simulink library "NNodeTether_cl"  (R2018b)
settings: Solver=VariableStepAuto  StartTime=0.0  StopTime=10.0  RelTol=1e-3
undefined symbols (not defined in the file): ini_Ri_o, ini_Vi_o, thr
libraries: tetherBuoyancyAndWeightNGreater2_ul x1, tetherInternalForcesNGreater2_ul x1, tetherDragForceNGreater2_ul x1
settings Model: Creator=asiddiq2  LastModifiedBy=mcobb

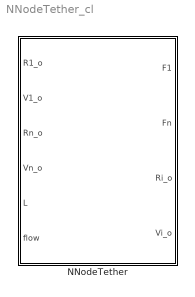
== system NNodeTether_cl ==
  NNodeTether : Subsystem

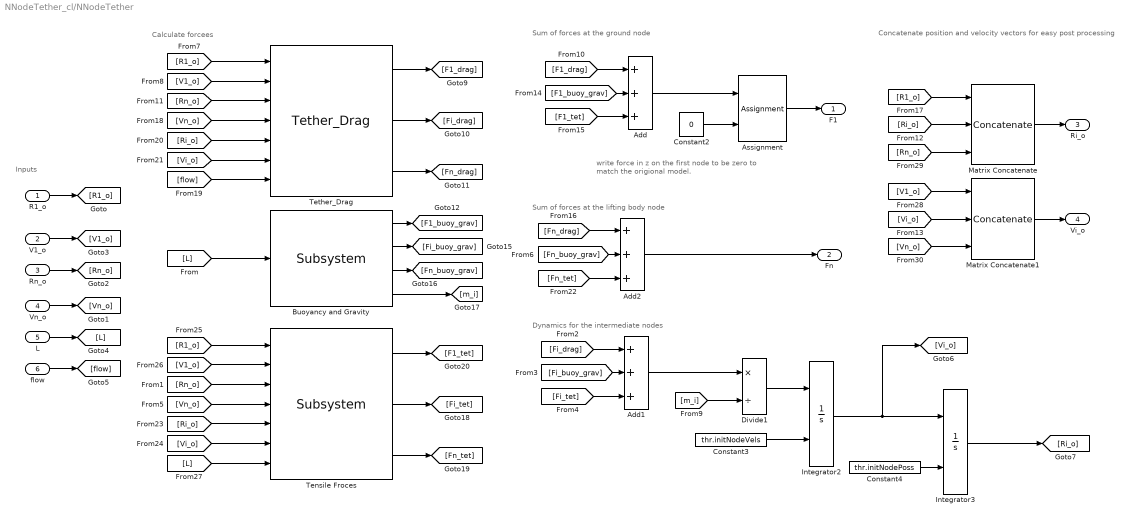
== system NNodeTether_cl/NNodeTether ==
  note: Concatenate position and velocity vectors for easy
      | post processing
  note: Calculate forcees
  note: Sum of forces at the lifting body node
  note: Dynamics for the intermediate nodes
  note: Sum of forces at the ground node
  note: write force in z on the first node to be zero
      | to match the origional model.
  note: Inputs
  R1_o : Inport
  V1_o : Inport  Port=2
  Rn_o : Inport  Port=3
  Vn_o : Inport  Port=4
  L : Inport  Port=5
  flow : Inport  Port=6
  Add : Sum  Inputs=+++
  Add1 : Sum  Inputs=+++
  Add2 : Sum  Inputs=+++
  Assignment : Assignment  NumberOfDimensions=2  DiagnosticForDimensions=Warning  IndexOptions=Index vector (dialog),Index vector (dialog)  Indices=3,1  OutputSizes=1,1
  Buoyancy and Gravity : tetherBuoyancyAndWeightNGreater2_ul/Subsystem  N=thr.N  dia_t=thr.diameter  rho_fluid=thr.fluidDensity  rho_tether=thr.density  g=thr.gravAccel
  Constant2 : Constant  Value=0
  Constant3 : Constant  Value=thr.initNodeVels
  Constant4 : Constant  Value=thr.initNodePoss
  Divide1 : Product  Inputs=*/
  Integrator2 : Integrator  InitialConditionSource=external  InitialCondition=ini_Vi_o
  Integrator3 : Integrator  InitialConditionSource=external  InitialCondition=ini_Ri_o
  Matrix Concatenate : Concatenate  NumInputs=3  Mode=Multidimensional array  ConcatenateDimension=2
  Matrix Concatenate1 : Concatenate  NumInputs=3  Mode=Multidimensional array  ConcatenateDimension=2
  Tensile Froces : tetherInternalForcesNGreater2_ul/Subsystem  N=thr.N  E=thr.youngsMod  dia_t=thr.diameter  mass=thr.vehicleMass  zeta=thr.dampingRatio
  Tether_Drag : tetherDragForceNGreater2_ul/Tether_Drag  Cd=thr.dragCoeff  rho_fluid=thr.fluidDensity  dia_t=thr.diameter
  F1 : Outport
  Fn : Outport  Port=2
  Ri_o : Outport  Port=3
  Vi_o : Outport  Port=4
  wires:
  R1_o/1 -> [R1_o]
  V1_o/1 -> [V1_o]
  Rn_o/1 -> [Rn_o]
  Vn_o/1 -> [Vn_o]
  L/1 -> [L]
  flow/1 -> [flow]
  [L] -> Buoyancy and Gravity/1
  [F1_buoy_grav] -> Add/2
  [F1_drag] -> Add/1
  [F1_tet] -> Add/3
  Assignment/1 -> F1/1
  Add/1 -> Assignment/1
  Constant2/1 -> Assignment/2
  Tether_Drag/1 -> [F1_drag]
  Tether_Drag/2 -> [Fi_drag]
  Tether_Drag/3 -> [Fn_drag]
  Buoyancy and Gravity/1 -> [F1_buoy_grav]
  Buoyancy and Gravity/2 -> [Fi_buoy_grav]
  Buoyancy and Gravity/3 -> [Fn_buoy_grav]
  Buoyancy and Gravity/4 -> [m_i]
  Tensile Froces/2 -> [Fi_tet]
  Tensile Froces/3 -> [Fn_tet]
  Tensile Froces/1 -> [F1_tet]
  [Fi_buoy_grav] -> Add1/2
  [Fi_tet] -> Add1/3
  [Fi_drag] -> Add1/1
  Add1/1 -> Divide1/1
  [m_i] -> Divide1/2
  Divide1/1 -> Integrator2/1
  Constant3/1 -> Integrator2/2
  Integrator2/1 -> [Vi_o], Integrator3/1
  Constant4/1 -> Integrator3/2
  Integrator3/1 -> [Ri_o]
  [Fn_drag] -> Add2/1
  [Fn_buoy_grav] -> Add2/2
  [Fn_tet] -> Add2/3
  Add2/1 -> Fn/1
  [R1_o] -> Tether_Drag/1
  [V1_o] -> Tether_Drag/2
  [Rn_o] -> Tether_Drag/3
  [Vn_o] -> Tether_Drag/4
  [Ri_o] -> Tether_Drag/5
  [Vi_o] -> Tether_Drag/6
  [flow] -> Tether_Drag/7
  [R1_o] -> Tensile Froces/1
  [Vn_o] -> Tensile Froces/4
  [Rn_o] -> Tensile Froces/3
  [Vi_o] -> Tensile Froces/6
  [Ri_o] -> Tensile Froces/5
  [V1_o] -> Tensile Froces/2
  [L] -> Tensile Froces/7
  [Rn_o] -> Matrix Concatenate/3
  [Ri_o] -> Matrix Concatenate/2
  [R1_o] -> Matrix Concatenate/1
  Matrix Concatenate/1 -> Ri_o/1
  [V1_o] -> Matrix Concatenate1/1
  Matrix Concatenate1/1 -> Vi_o/1
  [Vi_o] -> Matrix Concatenate1/2
  [Vn_o] -> Matrix Concatenate1/3
